simulink model "GDFLIB_FilterIIR1_BAM"  (Simulink 9.3)
settings: Solver=VariableStepAuto  StartTime=0.0  StopTime=10.0  RelTol=1e-3
settings Model: Creator=nxa18952  LastModifiedBy=nxa18952
settings DataIOCC: SaveFormat=Dataset  SignalLoggingSaveFormat=Dataset  ReturnWorkspaceOutputs=on
settings OptimizationCC: LifeSpan=auto
settings DebuggingCC: UnderspecifiedInitializationDetection=Simplified  MergeDetectMultiDrivingBlocksExec=error  FcnCallInpInsideContextMsg=error  SFUnexpectedBacktrackingDiag=error  SFNoUnconditionalDefaultTransitionDiag=error  SFExecutionAtInitializationDiag=warning  ArithmeticOperatorsInVariantConditions=error
settings HardwareCC: ProdBitPerPointer=64  ProdBitPerSizeT=64  ProdBitPerPtrDiffT=64  ProdLargestAtomicFloat=Float  ProdIntDivRoundTo=Zero  ProdEndianess=LittleEndian  ProdWordSize=64  ProdHWDeviceType=Intel->x86-64 (Windows64)
settings ModelReferenceCC: PropagateSignalLabelsOutOfModel=on
settings SFSimCC: SimUseLocalCustomCode=on
settings RTWCC: RTWUseLocalCustomCode=on
settings CodeAppCC: StateflowObjectComments=off
settings GRTTargetCC: TargetLangStandard=C99 (ISO)  CombineOutputUpdateFcns=on  GRTInterface=off
settings ConfigComp: CovMetricSettings=dwe  CovHtmlReporting=off  CovSaveCumulativeToWorkspaceVar=off  CovSaveSingleToWorkspaceVar=off  CovExternalEMLEnable=on

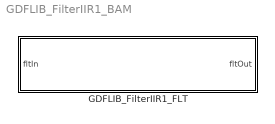
== system GDFLIB_FilterIIR1_BAM ==
  GDFLIB_FilterIIR1_FLT : Subsystem  TreatAsAtomicUnit=on  mask(GDFLIB_FilterIIR1_FLT){showStates=Hide (faster execution), fltB0=0, fltB1=0, fltA1=0}
      mask prompts: showStates "Show internal states"; fltB0 "fltB0 (B0 coefficient of the IIR1 filter in single precision floating-point format)"; fltB1 "fltB1 (B1 coefficient of the IIR1 filter in single precision floating-point format)"; fltA1 "fltA1 (A1 coefficient of the IIR1 filter in single precision floating-point format)"
      mask help: Direct form I first order IIR filter in single precision floating-point implementation. Refer to the AMMCLIB User's Guide for further details.
      mask init:
      | if ~evalin('base','exist(''tS8'',''var'')')
      |   if (2 ~= exist('SWLIBS_Typedefs.mat','file'))
      |       error('File SWLIBS_Typedefs.mat is not on the Matlab path. Please add the AMMCLIB "bam" folder in the Matlab Search Path.');
      |   else
      |       evalin('base', 'load(''SWLIBS_Typedefs.mat'')');
      |   end
      | end
      | if showStates == 1
      |     % hidden state variables
      |     if strcmp(get_param([gcb '/fltB0'], 'BlockType'), 'Inport')
      |         posblk = get_param(gcb, 'Position');
      | 
      |         pos = get_param(    [gcb, '/fltB0'], 'Position');
      |         orient = get_param( [gcb, '/fltB0'], 'Orientation');
      |         delete_block(       [gcb, '/fltB0']);
      |         add_block('built-in/Ground', [gcb, '/fltB0'], 'Position', pos, 'Orientation', orient);
      | 
      |         pos = get_param(    [gcb, '/fltB1'], 'Position');
      |         orient = get_param( [gcb, '/fltB1'], 'Orientation');
      |         delete_block(       [gcb, '/fltB1']);
      |         add_block('built-in/Ground', [gcb, '/fltB1'], 'Position', pos, 'Orientation', orient);
      | 
      |         pos = get_param(    [gcb, '/fltA1'], 'Position');
      |         orient = get_param( [gcb, '/fltA1'], 'Orientation');
      |         delete_block(       [gcb, '/fltA1']);
      |         add_block('built-in/Ground', [gcb, '/fltA1'], 'Position', pos, 'Orientation', orient);
      | 
      |         pos = get_param(    [gcb, '/fltFiltBufferX'], 'Position');
      |         orient = get_param( [gcb, '/fltFiltBufferX'], 'Orientation');
      |         delete_block(       [gcb, '/fltFiltBufferX']);
      |         add_block('built-in/Ground', [gcb, '/fltFiltBufferX'], 'Position', pos, 'Orientation', orient);
      | 
      |         pos = get_param(    [gcb, '/fltFiltBufferY'], 'Position');
      |         orient = get_param( [gcb, '/fltFiltBufferY'], 'Orientation');
      |         delete_block(       [gcb, '/fltFiltBufferY']);
      |         add_block('built-in/Ground', [gcb, '/fltFiltBufferY'], 'Position', pos, 'Orientation', orient);
      | 
      | 
      |         pos = get_param(    [gcb '/fltFiltBufferX_Out'], 'Position');
      |         orient = get_param( [gcb '/fltFiltBufferX_Out'], 'Orientation');
      |         delete_block(       [gcb '/fltFiltBufferX_Out']);
      |         add_block('built-in/Terminator', [gcb '/fltFiltBufferX_Out'], 'Position', pos, 'Orientation', orient);
      | 
      |         pos = get_param(    [gcb '/fltFiltBufferY_Out'], 'Position');
      |         orient = get_param( [gcb '/fltFiltBufferY_Out'], 'Orientation');
      |         delete_block(       [gcb '/fltFiltBufferY_Out']);
      |         add_block('built-in/Terminator', [gcb '/fltFiltBufferY_Out'], 'Position', pos, 'Orientation', orient);
      | 
      | 
      |         set_param([gcb '/fltIn'], 'Port', '1');
      | 
      |         set_param([gcb '/fltOut'], 'Port', '1');
      | 
      |         set_param(gcb,'MaskEnables',{'on','on','on','on'});
      | 
      |         if (posblk(4) - posblk(2)) > 50
      |           height = 50;
      |           set_param(gcb,'Position',[posblk(1), posblk(2), posblk(3), posblk(2)+height])
      |         end
      |     end
      | else
      |     % shown state variables
      |     if strcmp(get_param([gcb '/fltB0'], 'BlockType'), 'Ground')
      |         posblk = get_param(gcb, 'Position');
      | 
      |         pos = get_param(    [gcb, '/fltB0'], 'Position');
      |         orient = get_param( [gcb, '/fltB0'], 'Orientation');
      |         delete_block(       [gcb, '/fltB0']);
      |         add_block('built-in/Inport', [gcb, '/fltB0'], 'Position', pos, 'Orientation', orient, 'OutDataTypeStr', 'single');
      | 
      |         pos = get_param(    [gcb, '/fltB1'], 'Position');
      |         orient = get_param( [gcb, '/fltB1'], 'Orientation');
      |         delete_block(       [gcb, '/fltB1']);
      |         add_block('built-in/Inport', [gcb, '/fltB1'], 'Position', pos, 'Orientation', orient, 'OutDataTypeStr', 'single');
      | 
      |         pos = get_param(    [gcb, '/fltA1'], 'Position');
      |         orient = get_param( [gcb, '/fltA1'], 'Orientation');
      |         delete_block(       [gcb, '/fltA1']);
      |         add_block('built-in/Inport', [gcb, '/fltA1'], 'Position', pos, 'Orientation', orient, 'OutDataTypeStr', 'single');
      | 
      |         pos = get_param(    [gcb, '/fltFiltBufferX'], 'Position');
      |         orient = get_param( [gcb, '/fltFiltBufferX'], 'Orientation');
      |         delete_block(       [gcb, '/fltFiltBufferX']);
      |         add_block('built-in/Inport', [gcb, '/fltFiltBufferX'], 'Position', pos, 'Orientation', orient, 'OutDataTypeStr', 'single');
      | 
      |         pos = get_param(    [gcb, '/fltFiltBufferY'], 'Position');
      |         orient = get_param( [gcb, '/fltFiltBufferY'], 'Orientation');
      |         delete_block(       [gcb, '/fltFiltBufferY']);
      |         add_block('built-in/Inport', [gcb, '/fltFiltBufferY'], 'Position', pos, 'Orientation', orient, 'OutDataTypeStr', 'single');
      | 
      | 
      |         pos = get_param(    [gcb '/fltFiltBufferX_Out'], 'Position');
      |         orient = get_param( [gcb '/fltFiltBufferX_Out'], 'Orientation');
      |         delete_block(       [gcb '/fltFiltBufferX_Out']);
      |         add_block('built-in/Outport', [gcb '/fltFiltBufferX_Out'], 'Position', pos, 'Orientation', orient);
      | 
      |         pos = get_param(    [gcb '/fltFiltBufferY_Out'], 'Position');
      |         orient = get_param( [gcb '/fltFiltBufferY_Out'], 'Orientation');
      |         delete_block(       [gcb '/fltFiltBufferY_Out']);
      |         add_block('built-in/Outport', [gcb '/fltFiltBufferY_Out'], 'Position', pos, 'Orientation', orient);
      | 
      | 
      |         set_param([gcb '/fltIn'], 'Port', '1');
      |         set_param([gcb '/fltB0'], 'Port', '2');
      |         set_param([gcb '/fltB1'], 'Port', '3');
      |         set_param([gcb '/fltA1'], 'Port', '4');
      |         set_param([gcb '/fltFiltBufferX'], 'Port', '5');
      |         set_param([gcb '/fltFiltBufferY'], 'Port', '6');
      | 
      |         set_param([gcb '/fltOut'], 'Port', '1');
      |         set_param([gcb '/fltFiltBufferX_Out'], 'Port', '2');
      |         set_param([gcb '/fltFiltBufferY_Out'], 'Port', '3');
      | 
      |         set_param(gcb,'MaskEnables',{'on','off','off','off'});
      | 
      |         if (posblk(4) - posblk(2)) < 175
      |           height = 175;
      |           set_param(gcb,'Position',[posblk(1), posblk(2), posblk(3), posblk(2)+height])
      |         end
      |     end
      | end
      settings: RTWSystemCode=Inline
      mask TypeOptions showStates: Hide (faster execution) | Show (allows debugging; connect feedback loops manually)
      mask Callback showStates:
      | maskStr = get_param(gcb,'showStates');
      | if strcmp(maskStr,'Hide (faster execution)'),
      |     set_param(gcb,'MaskEnables',{'on','on','on','on'});
      | else
      |     set_param(gcb,'MaskEnables',{'on','off','off','off'});
      | end
      mask Display:
      | color('black');
      | pos = get_param(gcb, 'Position');
      | width = pos(3) - pos(1);
      | height = pos(4) - pos(2);
      | tX=width/2;
      | tY=height - 8;
      | color('black');
      | text(tX,tY, 'GDFLIB_FilterIIR1_FLT', 'horizontalAlignment', 'center');
      | if showStates == 2
      |   color('red');
      |   text(tX,tY - 20, ['debugging mode' char(13) char(10) '(limited performance)'], 'horizontalAlignment', 'center');
      | end

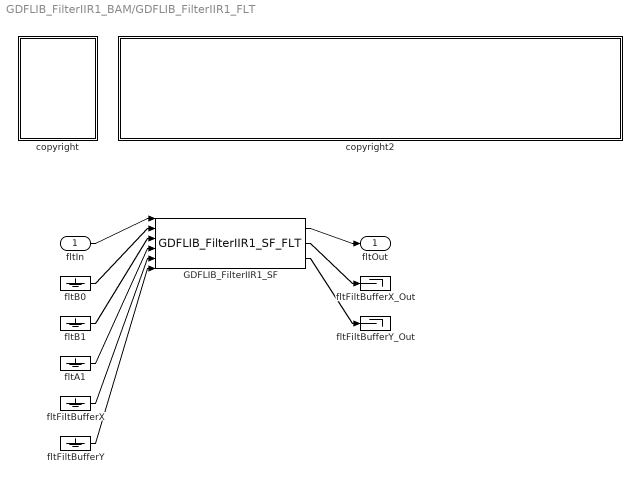
== system GDFLIB_FilterIIR1_BAM/GDFLIB_FilterIIR1_FLT ==
  fltIn : Inport  OutDataTypeStr=single
  GDFLIB_FilterIIR1_SF : S-Function  FunctionName=GDFLIB_FilterIIR1_SF_FLT  Parameters=showStates,fltB0,fltB1,fltA1  SFunctionDeploymentMode=off  EnableBusSupport=off
  copyright : Subsystem
      mask Display: text(10,90,'FILE:');text(10,75,'DESRIPTION:');text(10,60,'COPYRIGHT:');text(10,45,'VERSION:');text(10,30,'DATE:')
  copyright2 : Subsystem
      mask Display: text(10,90,'GDFLIB_FilterIIR1_BAM_FLT.mdl');text(10,75,'First order IIR filter.');text(10,60,'NXP 2020');text(10,45,'1.0');text(10,30,'18-Mar-2020');
  fltA1 : Ground
  fltB0 : Ground
  fltB1 : Ground
  fltFiltBufferX : Ground
  fltFiltBufferX_Out : Terminator
  fltFiltBufferY : Ground
  fltFiltBufferY_Out : Terminator
  fltOut : Outport
  wires:
  fltIn/1 -> GDFLIB_FilterIIR1_SF/1
  fltB0/1 -> GDFLIB_FilterIIR1_SF/2
  fltB1/1 -> GDFLIB_FilterIIR1_SF/3
  fltA1/1 -> GDFLIB_FilterIIR1_SF/4
  fltFiltBufferX/1 -> GDFLIB_FilterIIR1_SF/5
  fltFiltBufferY/1 -> GDFLIB_FilterIIR1_SF/6
  GDFLIB_FilterIIR1_SF/1 -> fltOut/1
  GDFLIB_FilterIIR1_SF/2 -> fltFiltBufferX_Out/1
  GDFLIB_FilterIIR1_SF/3 -> fltFiltBufferY_Out/1

== system GDFLIB_FilterIIR1_BAM/GDFLIB_FilterIIR1_FLT/copyright ==

== system GDFLIB_FilterIIR1_BAM/GDFLIB_FilterIIR1_FLT/copyright2 ==
